simulink library "CCM_FVT"  (R2024a)
settings: Solver=VariableStepAuto  StartTime=0.0  StopTime=10.0  RelTol=1e-3
undefined symbols (not defined in the file or in its folder): ACCM_facCCMLq_X_A, ACCM_facCCMLq_Y_A, ACCM_facLPFiDAct_X_rpm, ACCM_IdKp_X_rpm, ACCM_tiCurErrOvr_X_A, CCM_bRstIpartTrig_C, CCM_bRstPIMor_C, CCM_bRstPITrig_C, CCM_bUseCCMVolFFTrig_C, CCM_bUseUvw_flg, CCM_facAngleComp, CCM_facCCMKiUdTar_T, CCM_facCCMKiUqTar_T, CCM_facCCMKpUdTar_T, CCM_facCCMKpUqTar_T, CCM_facCCMLd_T, CCM_facCCMLq_T, CCM_facLPFiDAct_T, CCM_facLPFiQAct_T, CCM_iCurrDQRstIntgl_C, CCM_iDCurrAct_A, CCM_iDErrDeadZoneLo_C, CCM_iDErrDeadZoneUp_C, CCM_iQErrDeadZoneLo_C, CCM_iQErrDeadZoneUp_C, CCM_nRotCCMKpKi_A, CCM_nRotRstIntgl_C, CCM_nRotSpdLPFiDQAct_A, CCM_uDVoltTarMax_C, CCM_uDVoltTarMin_C, CCM_uDVoltTarMor_C, CCM_uDVoltTarTrig_C, CCM_uQVoltTarMax_C, CCM_uQVoltTarMin_C, CCM_uQVoltTarMor_C, CCM_uQVoltTarTrig_C, CDC_iQCurrAct_A, CDC_tqMotCurrTarMTPV_A, ENUM_IVTROPMODE_DTCYCTRL, IvtrM_vVehPCM2SpdKpKiTar_A, KCCM_BattVolFilTi_fac, KCCM_bRstCurErrorOverThd_C, KCCM_CurLoopPrd_t, KCCM_FwdMask_c, KCCM_IdKi_null, KCCM_IdKp_null, KCCM_IdKt_null, KCCM_IqKi_null, KCCM_IqKp_null, KCCM_IqKt_null, KCCM_PosnRange_deg, KCCM_tiCurErrOvr_C, KCCM_UdqASCEna_C, KCCM_UdqASCTagValue_C, KCCM_UdqASCTimesValue_C, KCCM_VdSp_V, KCCM_VdSpSwEna_flg, KCCM_VolMod_perc, KCCM_VqSp_V, KDSM_CurErrorThd2_value ... (+33)
libraries: simulink x10, GRC_Lib x6, FVTMCU_lib x2
(part 2 of 2)

== system CCM_FVT/CCM_FVT/CurrLoop/PI/IqPI ==
  note: The output is calculated as:
      | err = Setpoint-Value
      | result = K*err + Integral*CurLoopEna + Fwd
      | Integral = Integral + Ki*Tsam*err + Kt*Tsam*antiwindup
      | Tsam is the period of PI regulator.
  note: 0.000125
  "SpdFil " : Inport
  CurLoopActEna : Inport  Port=2
  IqCmd : Inport  Port=3
  IqFb : Inport  Port=4
  VqFwd : Inport  Port=5
  VqLim : Inport  Port=6
  Constant2 : Constant  Value=KCCM_FwdMask_c  OutDataTypeStr=single
  Iq_Regulator : Subsystem
  MCCM_IqKp_value : Lookup_n-D  NumberOfTableDimensions=1  BreakpointsForDimension1=ACCM_IdKp_X_rpm  Table=MCCM_IqKp_Y_value  ExtrapMethod=Clip  UseLastTableValue=on  InternalRulePriority=Speed  RndMeth=Simplest
  Product3 : Product  Inputs=**  RndMeth=Zero
  TM_Id_Ki : Constant  Value=KCCM_IqKi_null  OutDataTypeStr=single
  TM_Id_Kp : Constant  Commented=on  Value=KCCM_IqKp_null  OutDataTypeStr=single
  TM_Id_Kt : Constant  Value=KCCM_IqKt_null  OutDataTypeStr=single
  TM_Prd : Constant  Value=KCCM_CurLoopPrd_t  OutDataTypeStr=single
  Terminator : Terminator  Commented=on
  VqRef : Outport
  wires:
  Product3/1 -> Iq_Regulator/4(Fwd)
  Constant2/1 -> Product3/2
  VqFwd/1 -> Product3/1
  TM_Prd/1 -> Iq_Regulator/9(Prd)
  TM_Id_Kt/1 -> Iq_Regulator/8(Tt)
  TM_Id_Ki/1 -> Iq_Regulator/7(Ti)
  VqLim/1 -> Iq_Regulator/3(maxOutput)
  IqFb/1 -> Iq_Regulator/2(Feedback)
  IqCmd/1 -> Iq_Regulator/1(set point)
  Iq_Regulator/1(result) -> VqRef/1
  CurLoopActEna/1 -> Iq_Regulator/5(CurLoopEna)
  MCCM_IqKp_value/1 -> Iq_Regulator/6(Kp)
  TM_Id_Kp/1 -> Terminator/1
  "SpdFil "/1 -> MCCM_IqKp_value/1

== system CCM_FVT/CCM_FVT/CurrLoop/RCM/Subsystem ==
  "VCCM_VoltCmd_V " : Inport
  "VCCM_CurFb_A " : Inport  Port=2
  "Reset " : Inport  Port=3
  Constant : Constant  Value=KRCM_motorRs_value
  Constant2 : Constant  Value=KRCM_PIKp_value
  Constant3 : Constant  Value=KRCM_PIKi_value*KCCM_CurLoopPrd_t  OutDataTypeStr=single
  Logical Operator : Logic  Operator=NOT  AllPortsSameDT=off  OutDataTypeStr=boolean
  "PI " : Subsystem
  Product1 : Product
  Sum : Sum  Inputs=|+-  OutDataTypeStr=Inherit: Same as first input
  "Wrapp " : Subsystem
  "VRCM_RsvLrnAngle_rad " : Outport  VectorParamsAs1DForOutWhenUnconnected=off
  wires:
  "VCCM_VoltCmd_V "/1 -> Sum/1
  Constant2/1 -> "PI "/2(Kp)
  Product1/1 -> Sum/2
  Constant3/1 -> "PI "/3(Ki)
  Constant/1 -> Product1/1
  "VCCM_CurFb_A "/1 -> Product1/2
  Sum/1 -> "PI "/1(error)  "KRCM_VoltError_value"
  "PI "/1(Out) -> "Wrapp "/1(In1)
  "Wrapp "/1(Out2) -> "VRCM_RsvLrnAngle_rad "/1
  "Reset "/1 -> Logical Operator/1
  Logical Operator/1 -> "PI "/4("Reset ")

== system CCM_FVT/CCM_FVT/CurrLoop/VdqLim/VdFilter ==
  note: Description:
      | 1 order low pass filter. The constant value depends on the cut-off frequency,
  Measured : Inport  PortDimensions=1
  Add : Sum
  Constant : Constant  Value=KCCM_BattVolFilTi_fac  OutDataTypeStr=single
  Product : Product  OutDataTypeStr=single  RndMeth=Zero
  Subtract : Sum  Inputs=+-
  Unit Delay : UnitDelay  SampleTime=-1
  Filtered : Outport
  wires:
  Add/1 -> Unit Delay/1, Filtered/1
  Product/1 -> Add/1
  Constant/1 -> Product/2
  Subtract/1 -> Product/1
  Unit Delay/1 -> Add/2, Subtract/2
  Measured/1 -> Subtract/1

== system CCM_FVT/CCM_FVT/CurrLoop/VdqLim/VdFilter1 ==
  note: Description:
      | 1 order low pass filter. The constant value depends on the cut-off frequency,
  Measured : Inport  PortDimensions=1
  Add : Sum
  Constant : Constant  Value=KCCM_BattVolFilTi_fac  OutDataTypeStr=single
  Product : Product  RndMeth=Zero
  Subtract : Sum  Inputs=+-
  Unit Delay : UnitDelay  SampleTime=-1
  Filtered : Outport
  wires:
  Measured/1 -> Subtract/1
  Unit Delay/1 -> Subtract/2, Add/2
  Subtract/1 -> Product/1
  Constant/1 -> Product/2
  Product/1 -> Add/1
  Add/1 -> Filtered/1, Unit Delay/1

== system CCM_FVT/CCM_FVT/CurrLoop/ActCurrDQ/UvToDq/Clarke_Function ==
  PhaUCur : Inport  PortDimensions=1
  PhaVCur : Inport  Port=2  PortDimensions=1
  Constant4 : Constant  Value=0.57735  OutDataTypeStr=single
  Gain : Gain  Gain=2
  Product4 : Product  InputSameDT=on  RndMeth=Zero  OutDataTypeStr=Inherit: Same as first input
  Product5 : Product  InputSameDT=on  RndMeth=Zero  OutDataTypeStr=Inherit: Same as first input
  Sum3 : Sum  InputSameDT=on  OutDataTypeStr=Inherit: Same as first input
  IalphaFb : Outport  PortDimensions=1
  IbetaFb : Outport  Port=2  PortDimensions=1
  wires:
  PhaUCur/1 -> IalphaFb/1, Product4/1
  PhaVCur/1 -> Product5/2
  Product4/1 -> Sum3/1
  Product5/1 -> Gain/1
  Sum3/1 -> IbetaFb/1
  Constant4/1 -> Product4/2, Product5/1
  Gain/1 -> Sum3/2

== system CCM_FVT/CCM_FVT/CurrLoop/ActCurrDQ/UvToDq/Park_Function ==
  IalphaFb : Inport  PortDimensions=1
  IbetaFb : Inport  Port=2  PortDimensions=1
  Sin : Inport  Port=3  PortDimensions=1
  Cos : Inport  Port=4  PortDimensions=1
  Product{3,6..8} (4 alike) : Product  InputSameDT=on  RndMeth=Zero  OutDataTypeStr=Inherit: Same as first input
  Sum2 : Sum  InputSameDT=on  SaturateOnIntegerOverflow=on  OutDataTypeStr=Inherit: Same as first input
  Sum4 : Sum  Inputs=-+  InputSameDT=on  SaturateOnIntegerOverflow=on  OutDataTypeStr=Inherit: Same as first input
  IqFb : Outport  PortDimensions=1
  IdFb : Outport  Port=2  PortDimensions=1
  wires:
  IbetaFb/1 -> Product8/1, Product6/1
  Sin/1 -> Product6/2, Product7/2
  Product3/1 -> Sum2/1
  Product6/1 -> Sum2/2
  Product7/1 -> Sum4/1
  Product8/1 -> Sum4/2
  Cos/1 -> Product8/2, Product3/2
  IalphaFb/1 -> Product3/1, Product7/1
  Sum2/1 -> IdFb/1
  Sum4/1 -> IqFb/1

== system CCM_FVT/CCM_FVT/CurrLoop/ActCurrDQ/UvToDq/TriAgTbl ==
  Posn : Inport
  PosnRange : Inport  Port=2
  Product2 : Product  OutDataTypeStr=single  RndMeth=Zero
  Product3 : Product  OutDataTypeStr=single  RndMeth=Zero
  SinCos1 : Stateflow chart  TreatAsAtomicUnit=on
  sin1 : Lookup  InputValues=[0:1023]  Table=Sin_Table  LookUpMeth=Use Input Nearest  OutDataTypeStr=single  SaturateOnIntegerOverflow=off
  sin2 : Lookup  InputValues=[0:1023]  Table=Sin_Table  LookUpMeth=Use Input Nearest  OutDataTypeStr=single  SaturateOnIntegerOverflow=off
  Sin : Outport
  Cos : Outport  Port=2
  wires:
  Product2/1 -> Sin/1
  Product3/1 -> Cos/1
  SinCos1/1(Sin_theta) -> sin1/1
  SinCos1/2(SignSin) -> Product2/2
  sin1/1 -> Product2/1
  SinCos1/4(Cos_theta) -> sin2/1
  sin2/1 -> Product3/2
  SinCos1/3(SignCos) -> Product3/1
  Posn/1 -> SinCos1/1(Posn)
  PosnRange/1 -> SinCos1/2(PosnRange)

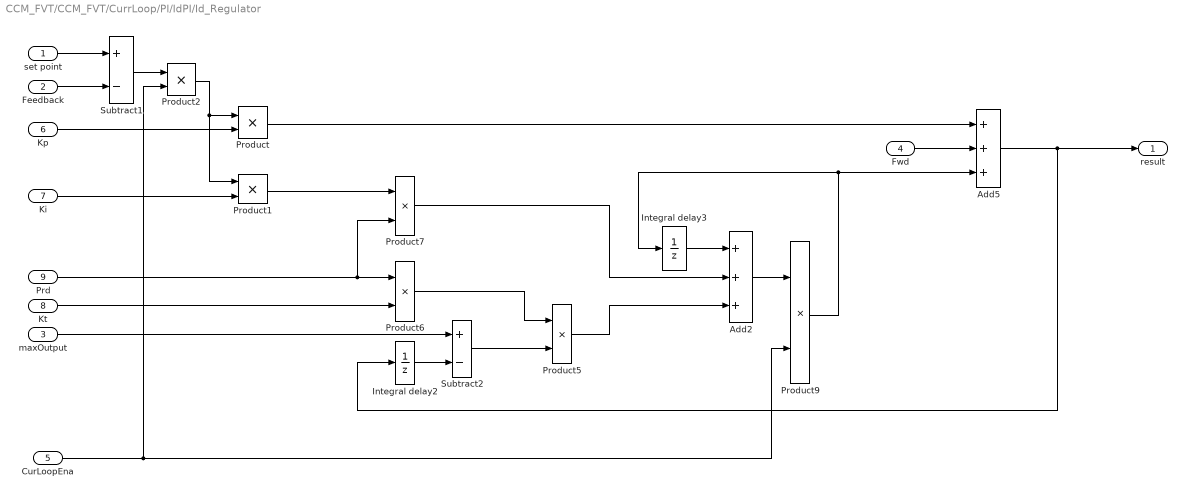
== system CCM_FVT/CCM_FVT/CurrLoop/PI/IdPI/Id_Regulator ==
  set point : Inport
  Feedback : Inport  Port=2
  maxOutput : Inport  Port=3
  Fwd : Inport  Port=4
  CurLoopEna : Inport  Port=5  PortDimensions=1
  Kp : Inport  Port=6  PortDimensions=1
  Ki : Inport  Port=7  PortDimensions=1
  Kt : Inport  Port=8  PortDimensions=1
  Prd : Inport  Port=9  PortDimensions=1
  Add2 : Sum  Inputs=+++
  Add5 : Sum  Inputs=+++
  Integral delay2 : UnitDelay  SampleTime=-1
  Integral delay3 : UnitDelay  SampleTime=-1
  Product{,1..2,5..7} (6 alike) : Product  RndMeth=Zero
  Product9 : Product  OutDataTypeStr=single  RndMeth=Zero
  Subtract1 : Sum  Inputs=+-
  Subtract2 : Sum  Inputs=+-
  result : Outport  OutDataTypeStr=single
  wires:
  Product2/1 -> Product1/1, Product/1
  Ki/1 -> Product1/2
  Product1/1 -> Product7/1
  Product6/1 -> Product5/1
  Add5/1 -> Integral delay2/1, result/1
  CurLoopEna/1 -> Product2/2, Product9/2
  Add2/1 -> Product9/1
  Fwd/1 -> Add5/2
  Product5/1 -> Add2/3
  Integral delay3/1 -> Add2/1
  Product9/1 -> Add5/3, Integral delay3/1
  Product/1 -> Add5/1
  Product7/1 -> Add2/2
  Kp/1 -> Product/2
  Kt/1 -> Product6/2
  Prd/1 -> Product7/2, Product6/1
  Subtract2/1 -> Product5/2
  Integral delay2/1 -> Subtract2/2
  maxOutput/1 -> Subtract2/1
  Feedback/1 -> Subtract1/2
  set point/1 -> Subtract1/1
  Subtract1/1 -> Product2/1

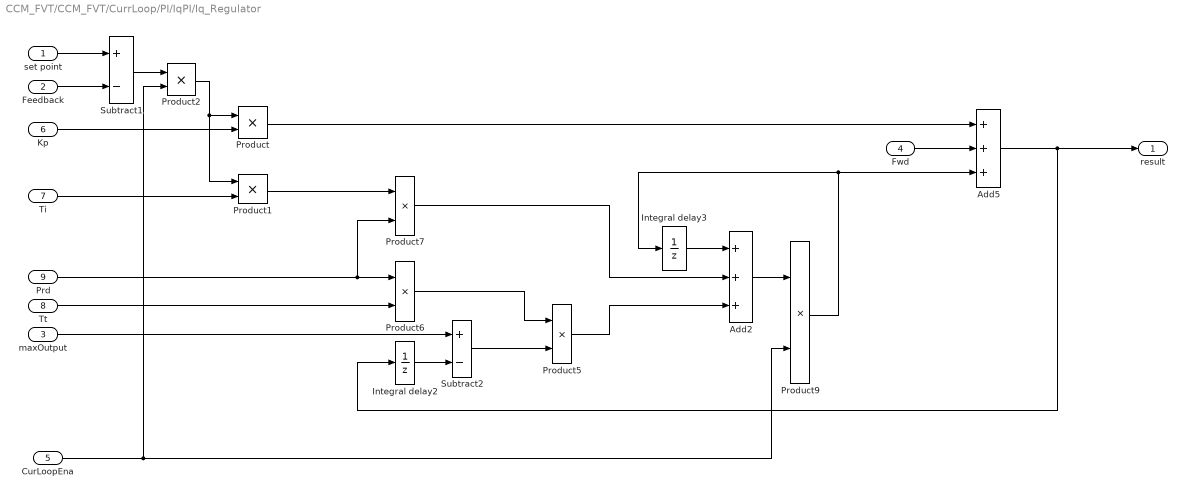
== system CCM_FVT/CCM_FVT/CurrLoop/PI/IqPI/Iq_Regulator ==
  set point : Inport
  Feedback : Inport  Port=2
  maxOutput : Inport  Port=3
  Fwd : Inport  Port=4
  CurLoopEna : Inport  Port=5  PortDimensions=1
  Kp : Inport  Port=6  PortDimensions=1
  Ti : Inport  Port=7  PortDimensions=1
  Tt : Inport  Port=8  PortDimensions=1
  Prd : Inport  Port=9  PortDimensions=1
  Add2 : Sum  Inputs=+++
  Add5 : Sum  Inputs=+++
  Integral delay2 : UnitDelay  SampleTime=-1
  Integral delay3 : UnitDelay  SampleTime=-1
  Product{,1..2,5..7} (6 alike) : Product  RndMeth=Zero
  Product9 : Product  OutDataTypeStr=single  RndMeth=Zero
  Subtract1 : Sum  Inputs=+-
  Subtract2 : Sum  Inputs=+-
  result : Outport  OutDataTypeStr=single
  wires:
  Product2/1 -> Product1/1, Product/1
  Subtract1/1 -> Product2/1
  Ti/1 -> Product1/2
  Product1/1 -> Product7/1
  Product6/1 -> Product5/1
  Add5/1 -> Integral delay2/1, result/1
  CurLoopEna/1 -> Product2/2, Product9/2
  Add2/1 -> Product9/1
  Fwd/1 -> Add5/2
  Product5/1 -> Add2/3
  Integral delay3/1 -> Add2/1
  Product9/1 -> Add5/3, Integral delay3/1
  Product/1 -> Add5/1
  Product7/1 -> Add2/2
  Kp/1 -> Product/2
  Tt/1 -> Product6/2
  Prd/1 -> Product7/2, Product6/1
  Subtract2/1 -> Product5/2
  Integral delay2/1 -> Subtract2/2
  maxOutput/1 -> Subtract2/1
  Feedback/1 -> Subtract1/2
  set point/1 -> Subtract1/1

== system CCM_FVT/CCM_FVT/CurrLoop/RCM/Subsystem/PI  ==
  error : Inport
  Kp : Inport  Port=2
  Ki : Inport  Port=3
  "Reset " : Inport  Port=4
  Add : Sum
  Delay : Delay  DelayLength=1  ExternalReset=Level
      settings: InputPortMap=u0,r5
  Product : Product  RndMeth=Simplest  OutDataTypeStr=Inherit: Same as first input
  Product1 : Product  RndMeth=Simplest  OutDataTypeStr=Inherit: Same as first input
  Sum : Sum  Inputs=|++  RndMeth=Simplest  SaturateOnIntegerOverflow=on  OutDataTypeStr=Inherit: Same as first input
  Out : Outport
  wires:
  error/1 -> Product1/2, Product/1
  Kp/1 -> Product1/1
  Ki/1 -> Product/2
  Sum/1 -> Out/1
  Product1/1 -> Sum/1
  Product/1 -> Add/1
  Delay/1 -> Add/2
  Add/1 -> Sum/2, Delay/1
  "Reset "/1 -> Delay/2

== system CCM_FVT/CCM_FVT/CurrLoop/RCM/Subsystem/Wrapp  ==
  In1 : Inport
  Bias : Bias  Bias=-2*pi  SaturateOnIntegerOverflow=off
  Bias1 : Bias  Bias=+2*pi  SaturateOnIntegerOverflow=off
  Switch : Switch  Criteria=u2 > Threshold  Threshold=2*pi  SaturateOnIntegerOverflow=off  InputSameDT=off
  Switch1 : Switch  Criteria=u2 > Threshold  Threshold=2*pi  SaturateOnIntegerOverflow=off  InputSameDT=off
  Out2 : Outport  VectorParamsAs1DForOutWhenUnconnected=off
  wires:
  Switch/1 -> Switch1/1
  Bias/1 -> Switch/1
  In1/1 -> Bias1/1, Bias/1, Switch/3, Switch/2
  Bias1/1 -> Switch1/2, Switch1/3
  Switch1/1 -> Out2/1

== stateflow chart CCM_FVT/CurrLoop/ActCurrDQ/UvToDq/TriAgTbl/SinCos1 ==
  (default) -> (junction 34) : {Etheta_fb = Posn;}
  (junction 34) -> (junction 36) [order 2] : [Etheta_fb<0]
  (junction 34) -> (junction 35) [order 1] : [Etheta_fb>=PosnRange]
  (junction 36) -> (junction 38) : {
      | Etheta_fb = Etheta_fb + PosnRange;
      | }
  (junction 34) -> (junction 39) [order 3]
  (junction 35) -> (junction 37) : {
      | Etheta_fb = Etheta_fb - PosnRange;
      | }
  (junction 38) -> (junction 39)
  (junction 37) -> (junction 39)
  (junction 39) -> (junction 23)
  (junction 23) -> (junction 24) [order 1] : [Etheta_fb>=0&&Etheta_fb<PosnRange/4]
  (junction 23) -> (junction 26) [order 2]
  (junction 24) -> (junction 25) : {
      | Sin_theta=Etheta_fb;
      | Cos_theta=PosnRange/4-1-Etheta_fb;
      | SignSin=1;
      | SignCos=1;
      | }
  (junction 26) -> (junction 27) [order 1] : [Etheta_fb>=PosnRange/4&&Etheta_fb<PosnRange/2]
  (junction 26) -> (junction 29) [order 2]
  (junction 27) -> (junction 28) : {
      | Sin_theta=PosnRange/2-1-Etheta_fb;
      | Cos_theta=Etheta_fb-PosnRange/4;
      | SignSin=1;
      | SignCos=-1;
      | }
  (junction 29) -> (junction 30) [order 1] : [Etheta_fb>=PosnRange/2&&Etheta_fb<PosnRange*3/4]
  (junction 29) -> (junction 32) [order 2] : {
      | Sin_theta=PosnRange-1-Etheta_fb;
      | Cos_theta=Etheta_fb-PosnRange*3/4;
      | SignSin=-1;
      | SignCos=1;
      | }
  (junction 30) -> (junction 31) : {
      | Sin_theta=Etheta_fb-PosnRange/2;
      | Cos_theta=PosnRange*3/4-1-Etheta_fb;
      | SignSin=-1;
      | SignCos=-1;
      | }
  (junction 31) -> (junction 32)
  (junction 28) -> (junction 31)
  (junction 25) -> (junction 28)
  (junction 32) -> (junction 33)
  data: Sin_theta output int16; SignSin output int16; SignCos output int16; Cos_theta output int16; Posn input; PosnRange input; Etheta_fb local int16

== stateflow chart CCM_FVT/CurrLoop/ASCCal/Subsystem1/Ramp ==
  (default) -> (junction 89)
  (junction 89) -> (junction 90) [order 1] : [enableTrajGen_flg == 0]
      | {intVd = Vd; intVq = Vq;}
  (junction 89) -> (junction 91) [order 2]
  (junction 90) -> (junction 163) : {
      | deltaVd = (targetValue- Vd) / times * 0.0001;
      | deltaVq = (targetValue - Vq) / times * 0.0001;
      | }
  (junction 91) -> (junction 151) [order 1] : [abs(intVd - targetValue) > abs(deltaVd) ||abs(intVq - targetValue) > abs(deltaVq) ]
  (junction 91) -> (junction 101) [order 2] : {
      | intVd = targetValue;
      | intVq = targetValue;
      | enASC_flg = 1;
      | }
  (junction 151) -> (junction 186) : {
      | intVd = intVd + deltaVd;
      | intVq = intVq + deltaVq;
      | }
  (junction 101) -> (junction 186)
  (junction 186) -> (junction 163)
  (junction 163) -> (junction 206)
  data: intVd output single; Vd input; Vq input; enableTrajGen_flg input; deltaVq local single; intVq output single; deltaVd local single; targetValue input; times input single; enASC_flg output boolean
